simulink model "test04"  (R2021a)
settings: Solver=VariableStepAuto  StartTime=0.0  StopTime=10  RelTol=1e-3
libraries: HORTISIM x5
settings Model: Creator=djoroya  LastModifiedBy=djoroya
settings DebuggingCC: UnconnectedInputMsg=none  UnconnectedOutputMsg=none  UnconnectedLineMsg=none

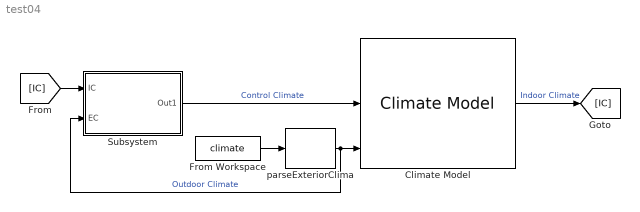
== system test04 ==
  Climate Model : HORTISIM/Climate/Models/Climate Model  hour0=0  G0=[0.05 0.0007]  T0=[273 273 273 273]+15  H=7  A_f=3200  A_c=3200  minWindows=0.1  lam_s=[2.5000 0.8500]  c_s=[1081 1081]  l_s=[0.1000 0.1000]  rhod_s=[2600 2500]  int_air_speed=0.5  alpha_i=0.1  alpha_c=0.05  tau_c=0.9  alpha_f=0.1  d_c=1.5  cd_c=8736  T_ss=285.15
      settings: SourceProductName=Horti Simulator
  From Workspace : FromWorkspace  VariableName=climate
  Subsystem : Subsystem
  parseExteriorClima : HORTISIM/Other  Functions/parseExteriorClima  SystemSampleTime=-1  VariantActivationTime=update diagram  Latency=0  AutoFrameSizeCalculation=off
      settings: SourceProductName=Horti Simulator
  wires:
  From Workspace/1 -> parseExteriorClima/1
  parseExteriorClima/1 -> Subsystem/2(EC), Climate Model/3  "Outdoor Climate"
  Climate Model/1 -> [IC]  "Indoor Climate"
  Subsystem/1(Out1) -> Climate Model/2  "Control Climate"
  [IC] -> Subsystem/1(IC)

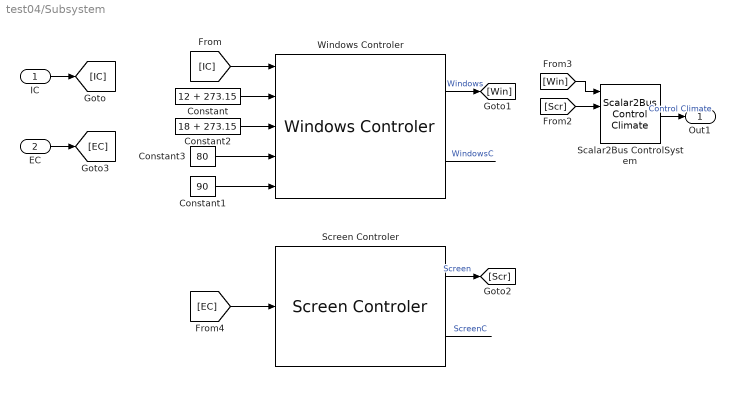
== system test04/Subsystem ==
  IC : Inport
  EC : Inport  Port=2
  Constant : Constant  Value=12 + 273.15
  Constant1 : Constant  Value=90
  Constant2 : Constant  Value=18 + 273.15
  Constant3 : Constant  Value=80
  Scalar2Bus ControlSystem : HORTISIM/Other  Functions/Scalar2Bus  Control Climate  SystemSampleTime=-1  VariantActivationTime=update diagram  Latency=0  AutoFrameSizeCalculation=off
      settings: SourceProductName=Horti Simulator
  Screen Controler : HORTISIM/Climate/Controls/Screen Controler  Radthreshold=200  velocity=0.33333  Power=0  gamma_max=0.3  beta=0.1
      settings: SourceProductName=Horti Simulator
  Windows Controler : HORTISIM/Climate/Controls/Windows Controler  Power=100  max_night=10  tau=600  RadThreshold=10  AR=10
      settings: SourceProductName=Horti Simulator
  Out1 : Outport
  wires:
  Constant2/1 -> Windows Controler/3
  Constant3/1 -> Windows Controler/4
  Windows Controler/2 -> ?  "WindowsC"
  Constant1/1 -> Windows Controler/5
  Constant/1 -> Windows Controler/2
  IC/1 -> [IC]
  [IC] -> Windows Controler/1
  Windows Controler/1 -> [Win]  "Windows"
  Screen Controler/1 -> [Scr]  "Screen"
  [Scr] -> Scalar2Bus ControlSystem/2
  [Win] -> Scalar2Bus ControlSystem/1
  Scalar2Bus ControlSystem/1 -> Out1/1  "Control Climate"
  EC/1 -> [EC]
  [EC] -> Screen Controler/1
  Screen Controler/2 -> ?  "ScreenC"
